simulink model "OptimalSol"  (R2019a)
settings: Solver=VariableStepAuto  StartTime=0.0  StopTime=tsim  MaxStep=1e-4  RelTol=1e-12  EnableMultiTasking=on
values from neighbouring files (symbols this model uses):
  Ap = 0.01    [aa_MAGLEV_changeSlope.m]
  bA = [A                 B1*Pi ... (first row only)    [aa_MAGLEV_changeSlope.m]    (also in optimizeL.m)
  bB2 = [B2; zeros((r+1)*q,m)]    [aa_MAGLEV_changeSlope.m]    (also in optimizeL.m)
  bC2 = [C2 zeros(p,(r+1)*q)]    [aa_MAGLEV_changeSlope.m]    (also in optimizeL.m)
  G0 = 0.015    [aa_MAGLEV_changeSlope.m]
  I0 = (1/Kb)*B0*G0    [aa_MAGLEV_changeSlope.m]
  Kb = 0.0015    [aa_MAGLEV_changeSlope.m]
  Kf = 9810    [aa_MAGLEV_changeSlope.m]
  Kfb = K    [aa_MAGLEV_changeSlope.m]
  L = inv(value(P))*value(Y)    [optimizeL.m]
  Lc = 0.1    [aa_MAGLEV_changeSlope.m]
  mc = 1000    [aa_MAGLEV_changeSlope.m]
  Nc = 2000    [aa_MAGLEV_changeSlope.m]
  Rc = 10    [aa_MAGLEV_changeSlope.m]
  V0 = I0*Rc    [aa_MAGLEV_changeSlope.m]
settings Model: Creator=alcasfra  LastModifiedBy=alcas
settings SolverCC: AlgebraicLoopSolver=LineSearch
settings DataIOCC: ReturnWorkspaceOutputs=off
settings OptimizationCC: LifeSpan=inf
settings DebuggingCC: SFUnexpectedBacktrackingDiag=warning  SFNoUnconditionalDefaultTransitionDiag=warning  ArithmeticOperatorsInVariantConditions=warning
settings SFSimCC: SimUseLocalCustomCode=off
settings RTWCC: RTWUseLocalCustomCode=off
settings CodeAppCC: StateflowObjectComments=on
settings GRTTargetCC: TargetLangStandard=C89/C90 (ANSI)  GeneratePreprocessorConditionals=Disable all
settings ConfigComp: CovMetricSettings=dw  CovHtmlReporting=on  CovSaveCumulativeToWorkspaceVar=on  CovSaveSingleToWorkspaceVar=on  CovExternalEMLEnable=off

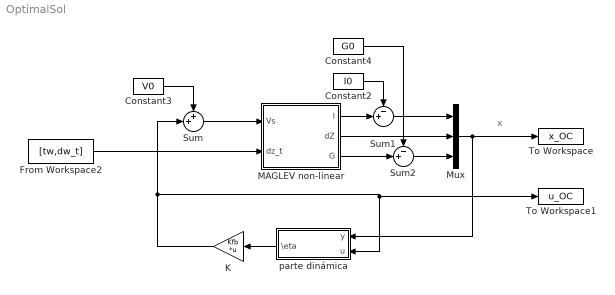
== system OptimalSol ==
  note: x
  Constant2 : Constant  Value=I0
  Constant3 : Constant  Value=V0
  Constant4 : Constant  Value=G0
  From Workspace2 : FromWorkspace  VariableName=[tw,dw_t]  SampleTime=0
  K : Gain  Gain=Kfb  Multiplication=Matrix(K*u)
  MAGLEV non-linear : Subsystem
  Mux : Mux  Inputs=3
  Sum : Sum  Inputs=++|
  Sum1 : Sum  Inputs=-+|
  Sum2 : Sum  Inputs=-+|
  To Workspace : ToWorkspace  VariableName=x_OC  SaveFormat=Structure With Time  SampleTime=-1
  To Workspace1 : ToWorkspace  VariableName=u_OC  SaveFormat=Structure With Time  SampleTime=-1
  parte dinámica : Subsystem
  wires:
  Sum/1 -> MAGLEV non-linear/1(Vs)
  Constant3/1 -> Sum/1
  MAGLEV non-linear/1(I) -> Sum1/2
  Sum1/1 -> Mux/1
  MAGLEV non-linear/3(G) -> Sum2/2
  Sum2/1 -> Mux/3
  Constant2/1 -> Sum1/1
  Constant4/1 -> Sum2/1
  MAGLEV non-linear/2(dZ) -> Mux/2
  Mux/1 -> parte dinámica/1(y), To Workspace/1
  parte dinámica/1(\eta) -> K/1
  K/1 -> Sum/2, parte dinámica/2(u), To Workspace1/1
  From Workspace2/1 -> MAGLEV non-linear/2(dz_t)

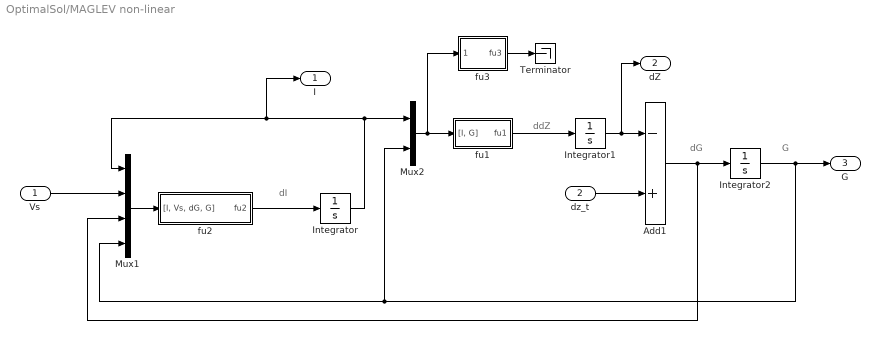
== system OptimalSol/MAGLEV non-linear ==
  note: G
  note: dG
  note: ddZ
  note: dI
  Vs : Inport
  dz_t : Inport  Port=2
  Add1 : Sum  Inputs=-+
  Integrator : Integrator  InitialCondition=I0
  Integrator1 : Integrator
  Integrator2 : Integrator  InitialCondition=G0
  Mux1 : Mux
  Mux2 : Mux  Inputs=2
  Terminator : Terminator
  fu1 : Subsystem
  fu2 : Subsystem
  fu3 : Subsystem
  I : Outport
  dZ : Outport  Port=2
  G : Outport  Port=3
  wires:
  fu3/1(fu3) -> Terminator/1
  Integrator/1 -> Mux2/1, I/1, Mux1/1
  fu1/1(fu1) -> Integrator1/1
  Integrator2/1 -> Mux2/2, Mux1/4, G/1
  Add1/1 -> Mux1/3, Integrator2/1
  dz_t/1 -> Add1/2
  Integrator1/1 -> dZ/1, Add1/1
  Mux2/1 -> fu3/1("[I, G]"), fu1/1("[I, G]")
  fu2/1(fu2) -> Integrator/1
  Mux1/1 -> fu2/1("[I, Vs, dG, G]")
  Vs/1 -> Mux1/2

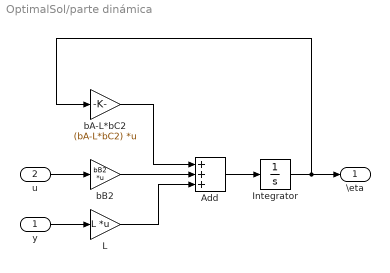
== system OptimalSol/parte dinámica ==
  y : Inport
  u : Inport  Port=2
  Add : Sum  Inputs=+++
  Integrator : Integrator
  L : Gain  Gain=L  Multiplication=Matrix(K*u)
  bA-L*bC2 : Gain  Gain=(bA-L*bC2)  Multiplication=Matrix(K*u)
  bB2 : Gain  Gain=bB2  Multiplication=Matrix(K*u)
  \eta : Outport
  wires:
  Integrator/1 -> \eta/1, bA-L*bC2/1
  bA-L*bC2/1 -> Add/1
  u/1 -> bB2/1
  Add/1 -> Integrator/1
  bB2/1 -> Add/2
  L/1 -> Add/3
  y/1 -> L/1

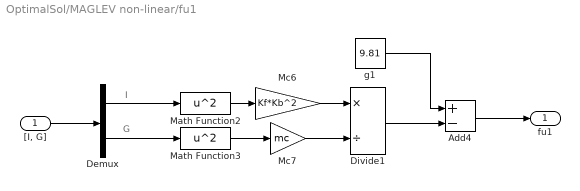
== system OptimalSol/MAGLEV non-linear/fu1 ==
  note: G
  note: I
  "[I, G]" : Inport
  Add4 : Sum  Inputs=+-
  Demux : Demux  Outputs=2
  Divide1 : Product  Inputs=*/
  Math Function2 : Math  Operator=square  SaturateOnIntegerOverflow=on
  Math Function3 : Math  Operator=square  SaturateOnIntegerOverflow=on
  Mc6 : Gain  Gain=Kf*Kb^2
  Mc7 : Gain  Gain=mc
  g1 : Constant  Value=9.81
  fu1 : Outport
  wires:
  g1/1 -> Add4/1
  Math Function2/1 -> Mc6/1
  Add4/1 -> fu1/1
  Demux/2 -> Math Function3/1
  "[I, G]"/1 -> Demux/1
  Demux/1 -> Math Function2/1
  Divide1/1 -> Add4/2
  Math Function3/1 -> Mc7/1
  Mc6/1 -> Divide1/1
  Mc7/1 -> Divide1/2

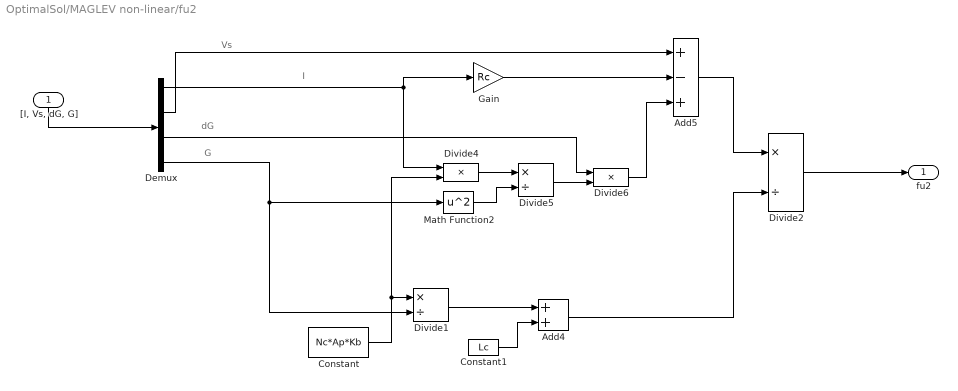
== system OptimalSol/MAGLEV non-linear/fu2 ==
  note: G
  note: dG
  note: Vs
  note: I
  "[I, Vs, dG, G]" : Inport
  Add4 : Sum
  Add5 : Sum  Inputs=+-+
  Constant : Constant  Value=Nc*Ap*Kb
  Constant1 : Constant  Value=Lc
  Demux : Demux
  Divide1 : Product  Inputs=*/
  Divide2 : Product  Inputs=*/
  Divide4 : Product  Inputs=**
  Divide5 : Product  Inputs=*/
  Divide6 : Product  Inputs=**
  Gain : Gain  Gain=Rc
  Math Function2 : Math  Operator=square  SaturateOnIntegerOverflow=on
  fu2 : Outport
  wires:
  Demux/1 -> Gain/1, Divide4/1
  Constant/1 -> Divide4/2, Divide1/1
  Divide2/1 -> fu2/1
  Constant1/1 -> Add4/2
  Demux/2 -> Add5/1
  Add5/1 -> Divide2/1
  Demux/4 -> Divide1/2, Math Function2/1
  Demux/3 -> Divide6/1
  "[I, Vs, dG, G]"/1 -> Demux/1
  Divide5/1 -> Divide6/2
  Divide1/1 -> Add4/1
  Add4/1 -> Divide2/2
  Math Function2/1 -> Divide5/2
  Divide4/1 -> Divide5/1
  Divide6/1 -> Add5/3
  Gain/1 -> Add5/2

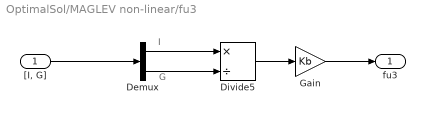
== system OptimalSol/MAGLEV non-linear/fu3 ==
  note: G
  note: I
  "[I, G]" : Inport
  Demux : Demux  Outputs=2
  Divide5 : Product  Inputs=*/
  Gain : Gain  Gain=Kb
  fu3 : Outport
  wires:
  Demux/2 -> Divide5/2
  Demux/1 -> Divide5/1
  Gain/1 -> fu3/1
  "[I, G]"/1 -> Demux/1
  Divide5/1 -> Gain/1
